simulink model "Pitch_for_speed_throttle_for_altitude"  (R2024b)
settings: Solver=ode4  StartTime=0.0  StopTime=200  FixedStep=0.05  MaxStep=30  RelTol=1e-3
undefined symbols (not defined in the file): utrim
libraries: simulink x1
settings Model: Creator=rzxha  LastModifiedBy=rzxha

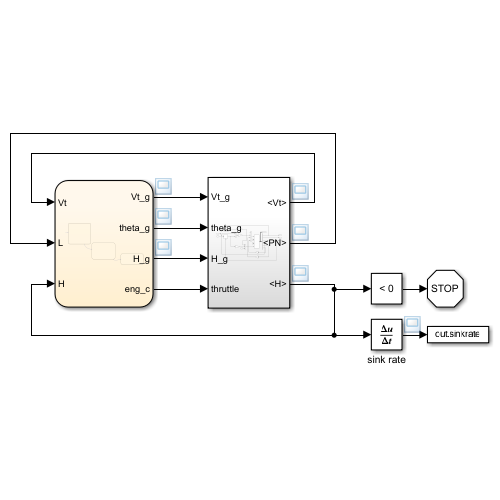
[thumbnail: Simulink's stored preview of the top-level diagram]
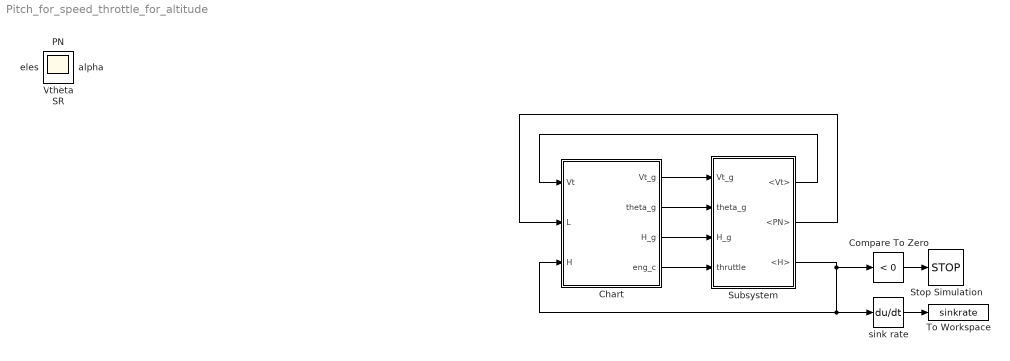
== system Pitch_for_speed_throttle_for_altitude ==
  Chart : Stateflow chart  TreatAsAtomicUnit=on
      settings: PortSchema="{\"entries\":[{\"content\":{\"sides\":[{\"content\":{\"connectorIds\":[\"In3\",\"In1\",\"In2\"]},\"type\":\"ConnectorPlacement.EquallySpacedRectSide\",\"uuid\":\"d20f7d6b-d091-49d1-bd40-2717f8cd9a8d\"},{\"content\":{\"connectorIds\":[\"Out4\",\"Out1\",\"Out3\",\"Out2\"],\"side\":\"RIGHT\"},\"type\":\"ConnectorPlacement.EquallySpacedRectSide\",\"uuid\":\"8772a0d8-7af3-469e-b51b-22dabe5fd991\"},{\"content\":{\"side\":\"TOP\"},\"type\":\"ConnectorPlacement.EquallySpacedRectSide\",\"uuid\":\"6dcf6d69-e3ca-4d70-96d9-b3e451e1b929\"},{\"content\":{\"side\":\"BOTTOM\"},\"type\":\"ConnectorPlacement.EquallySpacedRectSide\",\"uuid\":\"4ba253a7-eea1-4980-8d3e-b3eee014ca13\"}]},\"type\":\"ConnectorPlacement.EquallySpacedConnector\",\"uuid\":\"250d9512-bb95-400b-a793-090ba733a003\"}],\"packageUris\":[\"http://schema.mathworks.com/mf0/Connector/R2020b\"],\"version\":\"1.0\"}"
  Compare To Zero : simulink/Logic and Bit Operations/Compare To Zero  relop=<  OutDataTypeStr=boolean
  Stop Simulation : Stop
  Subsystem : Subsystem
  To Workspace : ToWorkspace  VariableName=sinkrate  SampleTime=-1
  sink rate : Derivative
  H : Scope
  PN : Scope
  SR : Scope
  Vt : Scope
  alpha : Scope
  eles : Scope
  theta : Scope
  wires:
  Compare To Zero/1 -> Stop Simulation/1
  Subsystem/3(<H>) -> Compare To Zero/1, sink rate/1, Chart/2(H)
  Chart/4(Vt_g) -> Subsystem/1(Vt_g)
  Chart/1(theta_g) -> Subsystem/2(theta_g)
  Chart/3(H_g) -> Subsystem/3(H_g)
  Chart/2(eng_c) -> Subsystem/4(thruttle)
  Subsystem/1(<Vt>) -> Chart/3(Vt)
  Subsystem/2(<PN>) -> Chart/1(L)
  sink rate/1 -> To Workspace/1

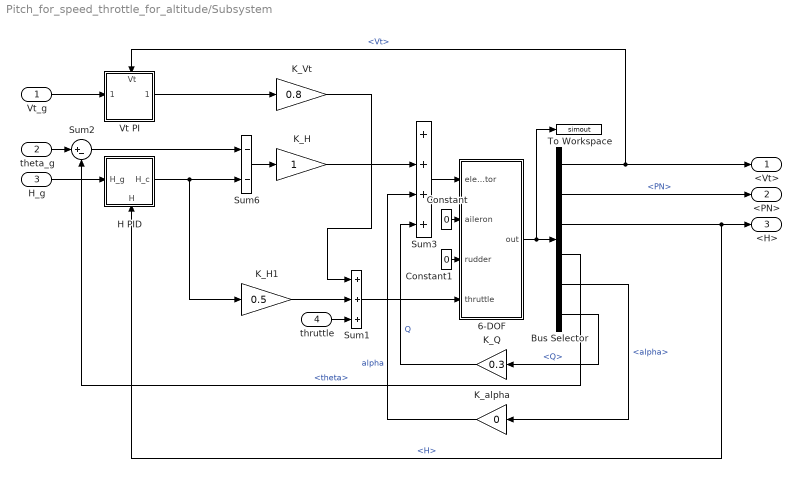
== system Pitch_for_speed_throttle_for_altitude/Subsystem ==
  Vt_g : Inport
  theta_g : Inport  Port=2
  H_g : Inport  Port=3
  thruttle : Inport  Port=4
  6-DOF : Subsystem
  Bus Selector : BusSelector  OutputSignals=Vt,PN,H,theta,alpha,Q
  Constant : Constant  Value=0
  Constant1 : Constant  Value=0
  H PID : Subsystem
      settings: PortSchema="{\"entries\":[{\"content\":{\"sides\":[{\"content\":{\"connectorIds\":[\"In1\"]},\"type\":\"ConnectorPlacement.EquallySpacedRectSide\",\"uuid\":\"28d2c1e8-6fce-41c2-b075-b38fe099c9fa\"},{\"content\":{\"connectorIds\":[\"Out1\"],\"side\":\"RIGHT\"},\"type\":\"ConnectorPlacement.EquallySpacedRectSide\",\"uuid\":\"4e2a0717-c77a-468e-a6aa-ad562fd9421a\"},{\"content\":{\"side\":\"TOP\"},\"type\":\"ConnectorPlacement.EquallySpacedRectSide\",\"uuid\":\"58ef56eb-719d-485c-87e2-46e257ded5a7\"},{\"content\":{\"connectorIds\":[\"In2\"],\"side\":\"BOTTOM\"},\"type\":\"ConnectorPlacement.EquallySpacedRectSide\",\"uuid\":\"bf9dfdfe-ea75-448e-b5f8-771b46288fbb\"}]},\"type\":\"ConnectorPlacement.EquallySpacedConnector\",\"uuid\":\"fdd112f0-5894-49ca-b631-3cb1072df4c6\"}],\"packageUris\":[\"http://schema.mathworks.com/mf0/Connector/R2020b\"],\"version\":\"1.0\"}"
  K_H : Gain
  K_H1 : Gain  Gain=0.5
  K_Q : Gain  Gain=0.3
  K_Vt : Gain  Gain=0.8
  K_alpha : Gain  Gain=0
  Sum1 : Sum  Inputs=+++
  Sum2 : Sum  Inputs=|+-
  Sum3 : Sum  Inputs=++++
  Sum6 : Sum  Inputs=--
  To Workspace : ToWorkspace  VariableName=simout  SampleTime=-1
  Vt PI : Subsystem
      settings: PortSchema="{\"entries\":[{\"content\":{\"sides\":[{\"content\":{\"connectorIds\":[\"In1\"]},\"type\":\"ConnectorPlacement.EquallySpacedRectSide\",\"uuid\":\"28d2c1e8-6fce-41c2-b075-b38fe099c9fa\"},{\"content\":{\"connectorIds\":[\"Out1\"],\"side\":\"RIGHT\"},\"type\":\"ConnectorPlacement.EquallySpacedRectSide\",\"uuid\":\"4e2a0717-c77a-468e-a6aa-ad562fd9421a\"},{\"content\":{\"connectorIds\":[\"In2\"],\"side\":\"TOP\"},\"type\":\"ConnectorPlacement.EquallySpacedRectSide\",\"uuid\":\"58ef56eb-719d-485c-87e2-46e257ded5a7\"},{\"content\":{\"side\":\"BOTTOM\"},\"type\":\"ConnectorPlacement.EquallySpacedRectSide\",\"uuid\":\"bf9dfdfe-ea75-448e-b5f8-771b46288fbb\"}]},\"type\":\"ConnectorPlacement.EquallySpacedConnector\",\"uuid\":\"fdd112f0-5894-49ca-b631-3cb1072df4c6\"}],\"packageUris\":[\"http://schema.mathworks.com/mf0/Connector/R2020b\"],\"version\":\"1.0\"}"
  <Vt> : Outport
  <PN> : Outport  Port=2
  <H> : Outport  Port=3
  wires:
  6-DOF/1(out) -> Bus Selector/1, To Workspace/1
  K_Q/1 -> Sum3/4  "Q"
  Bus Selector/6 -> K_Q/1  "<Q>"
  Sum6/1 -> K_H/1
  Bus Selector/5 -> K_alpha/1  "<alpha>"
  Constant1/1 -> 6-DOF/3(rudder)
  theta_g/1 -> Sum2/1
  Sum3/1 -> 6-DOF/1(elevator)
  H_g/1 -> H PID/1(H_g)
  Bus Selector/4 -> Sum2/2  "<theta>"
  K_alpha/1 -> Sum3/3  "alpha"
  K_H/1 -> Sum3/2
  Bus Selector/1 -> <Vt>/1, Vt PI/2(Vt)  "<Vt>"
  K_Vt/1 -> Sum1/1
  Bus Selector/2 -> <PN>/1  "<PN>"
  Vt PI/1(Vt_c) -> K_Vt/1
  Constant/1 -> 6-DOF/2(aileron)
  Bus Selector/3 -> H PID/2(H), <H>/1  "<H>"
  Vt_g/1 -> Vt PI/1(Vt_g)
  H PID/1(H_c) -> K_H1/1, Sum6/2
  Sum1/1 -> 6-DOF/4(thruttle)
  thruttle/1 -> Sum1/3
  K_H1/1 -> Sum1/2
  Sum2/1 -> Sum6/1

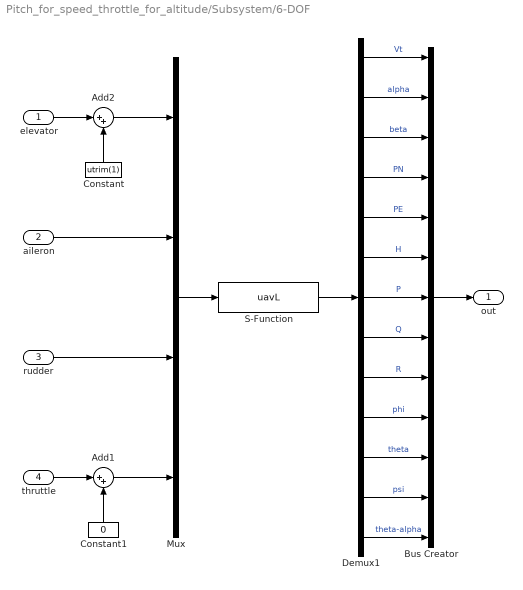
== system Pitch_for_speed_throttle_for_altitude/Subsystem/6-DOF ==
  elevator : Inport
  aileron : Inport  Port=2
  rudder : Inport  Port=3
  thruttle : Inport  Port=4
  Add1 : Sum  Inputs=|++
  Add2 : Sum  Inputs=|++
  Bus Creator : BusCreator  Inputs=13
  Constant : Constant  Value=utrim(1)
  Constant1 : Constant  Value=0
  Demux1 : Demux  Outputs=13
  Mux : Mux
  S-Function : S-Function  FunctionName=uavL  SFunctionDeploymentMode=off  EnableBusSupport=off
  out : Outport
  wires:
  Demux1/8 -> Bus Creator/8  "Q"
  elevator/1 -> Add2/1
  aileron/1 -> Mux/2
  Constant1/1 -> Add1/2
  Demux1/6 -> Bus Creator/6  "H"
  Constant/1 -> Add2/2
  thruttle/1 -> Add1/1
  Add1/1 -> Mux/4
  rudder/1 -> Mux/3
  Add2/1 -> Mux/1
  Mux/1 -> S-Function/1
  S-Function/1 -> Demux1/1
  Demux1/11 -> Bus Creator/11  "theta"
  Demux1/1 -> Bus Creator/1  "Vt"
  Demux1/13 -> Bus Creator/13  "theta-alpha"
  Demux1/2 -> Bus Creator/2  "alpha"
  Demux1/3 -> Bus Creator/3  "beta"
  Demux1/4 -> Bus Creator/4  "PN"
  Demux1/5 -> Bus Creator/5  "PE"
  Demux1/7 -> Bus Creator/7  "P"
  Demux1/9 -> Bus Creator/9  "R"
  Demux1/10 -> Bus Creator/10  "phi"
  Demux1/12 -> Bus Creator/12  "psi"
  Bus Creator/1 -> out/1

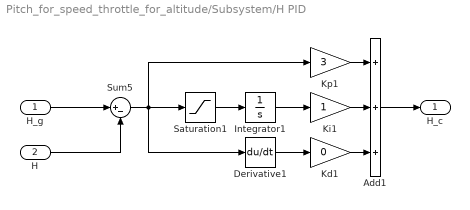
== system Pitch_for_speed_throttle_for_altitude/Subsystem/H PID ==
  H_g : Inport
  H : Inport  Port=2
  Add1 : Sum  Inputs=+++
  Derivative1 : Derivative
  Integrator1 : Integrator
  Kd1 : Gain  Gain=0
  Ki1 : Gain
  Kp1 : Gain  Gain=3
  Saturation1 : Saturate
  Sum5 : Sum  Inputs=|+-
  H_c : Outport
  wires:
  Derivative1/1 -> Kd1/1
  Ki1/1 -> Add1/2
  Integrator1/1 -> Ki1/1
  Add1/1 -> H_c/1
  Saturation1/1 -> Integrator1/1
  Kd1/1 -> Add1/3
  Kp1/1 -> Add1/1
  Sum5/1 -> Derivative1/1, Saturation1/1, Kp1/1
  H_g/1 -> Sum5/1
  H/1 -> Sum5/2

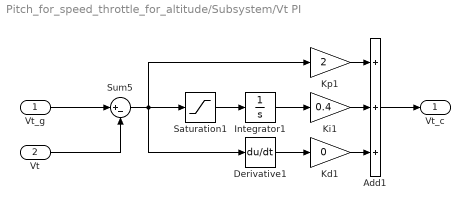
== system Pitch_for_speed_throttle_for_altitude/Subsystem/Vt PI ==
  Vt_g : Inport
  Vt : Inport  Port=2
  Add1 : Sum  Inputs=+++
  Derivative1 : Derivative
  Integrator1 : Integrator
  Kd1 : Gain  Gain=0
  Ki1 : Gain  Gain=0.4
  Kp1 : Gain  Gain=2
  Saturation1 : Saturate
  Sum5 : Sum  Inputs=|+-
  Vt_c : Outport
  wires:
  Derivative1/1 -> Kd1/1
  Ki1/1 -> Add1/2
  Integrator1/1 -> Ki1/1
  Add1/1 -> Vt_c/1
  Saturation1/1 -> Integrator1/1
  Kd1/1 -> Add1/3
  Kp1/1 -> Add1/1
  Sum5/1 -> Derivative1/1, Saturation1/1, Kp1/1
  Vt_g/1 -> Sum5/1
  Vt/1 -> Sum5/2

== stateflow chart Pitch_for_speed_throttle_for_altitude/Chart ==
  state level
    entry:
    theta_g = 2.340;
    eng_c = 36.169;
    H2 = 2; H1 = 55;
    path2 = 1; path1 = 3.5;
    %L2 = H2 / tan(deg2rad(path2));
    L2 = 114.580;
    %L1 = L2 + (H1 - H2) / tan(deg2rad(path1));
    L1 = 981.122;
    during:
    H_g = H1;
    Vt_g = Vt;
    exit:
  state dive
    entry:
    theta_g = -1.158;
    eng_c = 5;
    Vt_slope = (Vt - 18) / (H1 - H2);
    Vt_0 = Vt;
    during:
    H_g = H2 + (-L - L2) * tan(deg2rad(path1));
    Vt_g = Vt_0 - Vt_slope * (H1 - H);
    exit:
  state ballon
    entry:
    theta_g = 4; eng_c = 0;
    during:
    H_g = -L * tan(deg2rad(path2));
    %H_g = H;
    Vt_g = 17;
    exit:
  (default) -> level
  level -> dive : [L>-L1]
  dive -> ballon : [L>-L2]
  data: theta_g output; eng_c output; H_g output; L input; L2 local; L1 local; H1 local; H2 local; path2 local; path1 local; H input; Vt input; Vt_g output; Vt_0 local; Vt_slope local
